simulink model "BMS_V4"  (R2017b)
settings: Solver=FixedStepDiscrete  StartTime=0.0  StopTime=inf  FixedStep=BASETIME  RelTol=1e-3  EnableMultiTasking=on
values from neighbouring files (symbols this model uses):
  AKT_BALANCE = uint16(8)    [BMS_V4_config.m]
  BALANCE = uint16(4)    [BMS_V4_config.m]
  BALANCE_RESISTOR = int32(5)    [BMS_V4_config.m]
  BALANCE_VEC = uint16(8)    [BMS_V4_config.m]
  CELL_SOC = uint16(7)    [BMS_V4_config.m]
  CELL_STATE = uint16(3)    [BMS_V4_config.m]
  CELL_TEMPERATURE = uint16(6)    [BMS_V4_config.m]
  CELL_VOLTAGE = uint16(5)    [BMS_V4_config.m]
  CELLACTBITFIELD = hex2dec('300')    [BMS_V4_config.m]
  CELLDEACTBITFIELD = hex2dec('100')    [BMS_V4_config.m]
  CELLT_BURST = uint16(6)    [BMS_V4_config.m]
  CELLV_BURST = uint16(5)    [BMS_V4_config.m]
  CLK_CYC_timer_1 = 586    [BMS_V4_config.m]
  CLK_CYC_timer_2 = 5860    [BMS_V4_config.m]
  CLK_CYC_timer_3 = 280    [BMS_V4_config.m]
  CLK_CYC_timer_4 = 586*100    (= 58600)    [BMS_V4_config.m]
  CLK_CYC_timer_5 = 5800*2    (= 11600)    [BMS_V4_config.m]
  CLK_CYC_timer_6 = 320    [BMS_V4_config.m]
  CN_CELLS = int32(40*3600)    [BMS_V4_config.m]
  CONTACTOR = uint16(1)    [BMS_V4_config.m]
  CONTACTOR_LOCKED = uint16(0)    [BMS_V4_config.m]
  CONTACTOR_UNLOCKED = uint16(1)    [BMS_V4_config.m]
  DEBUG_SEND_STATES = uint16(hex2dec('01'))    [BMS_V4_config.m]
  DELTA_SOC_BALANCE = int32(5*1e6)    [BMS_V4_config.m]
  DELTA_SOC_BALANCE_OFF = int32(1*1e5)    [BMS_V4_config.m]
  DETERMINE_MODEL_PARAMETER_ACT = uint16(100)    [BMS_V4_config.m]
  DETERMINE_MODEL_PARAMETER_SCC = uint16(101)    [BMS_V4_config.m]
  ERROR = uint16(1)    [BMS_V4_config.m]
  EXTERN_SIGNALS = uint16(1)    [BMS_V4_config.m]
  FREQUENCY_STEPS = uint16([25 50 75 100 150 250 500 750                                      1000 1500 2500 5000 7500                                      10010 10015 10025 10050 10075                                      10100 10150 10250 10500 10750                                      11000 11500])    [BMS_V4_config.m]
  GET_IMAG_PART_MFC = uint16(9)    [BMS_V4_config.m]
  GET_IMAG_PART_MSF = uint16(4)    [BMS_V4_config.m]
  GET_REAL_PART_MFC = uint16(8)    [BMS_V4_config.m]
  GET_REAL_PART_MSF = uint16(3)    [BMS_V4_config.m]
  IMU = uint16(7)    [BMS_V4_config.m]
  IMU_AMP_OFF = uint16(5)    [BMS_V4_config.m]
  IMU_DATA_READ_LOCUS_ACT = uint16(6)    [BMS_V4_config.m]
  IMU_DATA_READ_LOCUS_SCC = uint16(7)    [BMS_V4_config.m]
  IMU_DEBUG = uint16(9)    [BMS_V4_config.m]
  IMU_GET_DATA_MFC = uint16(8)    [BMS_V4_config.m]
  IMU_GET_DATA_MSF = uint16(3)    [BMS_V4_config.m]
  IMU_OFFSET_POLLING = uint16(11)    [BMS_V4_config.m]
  IMU_POLLING = uint16(2)    [BMS_V4_config.m]
  IMU_POWER = uint16(10)    [BMS_V4_config.m]
  IMU_SEND_IMAG = uint16(11)    [BMS_V4_config.m]
  IMU_SEND_REAL = uint16(10)    [BMS_V4_config.m]
  INDEX_IMAGPART = uint16(2)    [BMS_V4_config.m]
  INDEX_REALPART = uint16(1)    [BMS_V4_config.m]
  INFO = uint16(2)    [BMS_V4_config.m]
  INIT_OFFSET_AMPLITUDE = uint16(2)    [BMS_V4_config.m]
  LINE_CURRENT = uint16(3)    [BMS_V4_config.m]
  LINE_CURRENT_CANA = uint16(4)    [BMS_V4_config.m]
  LINE_CURRENT_SWITCH_THRESHOLD = int32(2*1e6)    [BMS_V4_config.m]
  NUM_OF_CELLS = uint16(16)    [BMS_V4_config.m]
  NUM_OF_FREQUENCIES_PSO = uint16(14)    [BMS_V4_config.m]
  NUM_OF_LINES = uint16(1)    [BMS_V4_config.m]
  NUM_OF_PARAMETER = single(5)    [BMS_V4_config.m]
  NUM_OF_SOC_POINTS = uint16(110)    [BMS_V4_config.m]
  P_L_BOUND = single([0.05;0.01;0.1;0.01;0.1])    [BMS_V4_config.m]
  P_U_BOUND = single([0.50;0.20;0.9;0.06;60])    [BMS_V4_config.m]
  PARA_ACT_SEND = uint16(101)    [BMS_V4_config.m]
  PARA_DATA_STORE_ACT = uint16(8)    [BMS_V4_config.m]
  PARA_DATA_STORE_SCC = uint16(9)    [BMS_V4_config.m]
  PARA_SCC_SEND = uint16(102)    [BMS_V4_config.m]
  PARTICLE_INIT = single(create_startparticle(P_L_BOUND,P_U_BOUND,NUM_OF_PARTICLE))    [BMS_V4_config.m]
  POLACT = hex2dec('00000BFF')    [BMS_V4_config.m]
  POLDEACT = hex2dec('000008FF')    [BMS_V4_config.m]
  PSO_PARA_DEBUG = uint16(13)    [BMS_V4_config.m]
  REQUEST_SOC_REF = uint16(1000)    [BMS_V4_config.m]
  SCALE_FACTOR_CH1 = single(0.66666666)    [BMS_V4_config.m]
  SCALE_FACTOR_CH2 = single(0.66666666)    [BMS_V4_config.m]
  SEND_CELL_SOC_ABS = uint16(199)    [BMS_V4_config.m]
  SHUT_DOWN_BALANCE_OFF = uint16(3)    [BMS_V4_config.m]
  SHUT_DOWN_BALANCE_ON = uint16(2)    [BMS_V4_config.m]
  START_IMU_MSL = uint16(3)    [BMS_V4_config.m]
  START_IMU_SCC = uint16(1)    [BMS_V4_config.m]
  SWITCH_IMU_OFF = uint16(2)    [BMS_V4_config.m]
  SWITCH_IMU_ON = uint16(1)    [BMS_V4_config.m]
  SWITCH_IMU_ON_OFF = uint16(4)    [BMS_V4_config.m]
  SYSTEM_DEBUG = uint16(12)    [BMS_V4_config.m]
  TIMEOUT_CANA = uint32(5000)    [BMS_V4_config.m]
  TIMEOUT_GATEWAY = uint32(500)    [BMS_V4_config.m]
  TS_SOC = single(0.010)    [BMS_V4_config.m]
  WARNING = uint16(2)    [BMS_V4_config.m]
libraries: c280xlib x44, c2833xlib x5, simulink x2, c2000lib x1, idelinklib_common x1
(part 3 of 8)

== matlab function BMS_V4/FunctionCall_CANB_RX/handle_cellV_burst/cellV_proceeding ==
  data: msg input; NUM_OF_CELLS parameter; cell_voltages data_store_memory; next_gateway_request data_store_memory; gateway_request data_store_memory; CELLV_BURST parameter
function cellV_proceedng(msg,NUM_OF_CELLS, CELLV_BURST)

global cell_voltages;
global next_gateway_request;
global gateway_request;

x1      = uint16(bitand(uint32(hex2dec('0000FFFF')),msg(1)));
line_nr = uint16(bitand(uint16(hex2dec('00FF')),x1))+uint16(1);
cell_nr = uint16(bitand(uint16(hex2dec('00FF')),bitshift(x1,-8)))+uint16(1);
% cell number and line number starting with zero from Gateway
volt1   = uint16(bitand(uint32(hex2dec('0000FFFF')),bitshift(msg(1),-16)));
volt2   = uint16(bitand(uint32(hex2dec('0000FFFF')),bitshift(msg(2),-0)));
volt3   = uint16(bitand(uint32(hex2dec('0000FFFF')),bitshift(msg(2),-16)));

if (cell_nr + uint16(1)) > NUM_OF_CELLS % last msg with only one voltages
    cell_voltages(cell_nr, line_nr) = uint16(volt1); 
%     gateway_request(CELLV_BURST) = false;
    next_gateway_request=true;
elseif (cell_nr + uint16(2)) > NUM_OF_CELLS % last msg with only two voltages in msg
    cell_voltages(cell_nr, line_nr) = uint16(volt1); 
    cell_voltages(cell_nr+uint16(1),line_nr) = uint16(volt2);
%     gateway_request(CELLV_BURST) = false;
   next_gateway_request=true;
elseif (cell_nr + uint16(3)) > NUM_OF_CELLS % last msg with three voltages
    cell_voltages(cell_nr          , line_nr) = uint16(volt1); 
    cell_voltages(cell_nr+uint16(1), line_nr) = uint16(volt2);
    cell_voltages(cell_nr+uint16(2), line_nr) = uint16(volt3);
%     gateway_request(CELLV_BURST) = false;
    next_gateway_request=true;
else % more msg
    cell_voltages(cell_nr          , line_nr) = uint16(volt1); 
    cell_voltages(cell_nr+uint16(1), line_nr) = uint16(volt2);
    cell_voltages(cell_nr+uint16(2), line_nr) = uint16(volt3);
end

== matlab function BMS_V4/FunctionCalll_CANB_send/Send_gateway_request_control ==
  data: contactor_enable output; CAN_contactor_low output; CAN_contactor_high output; info_enable output; CAN_info_low output; CAN_info_high output; line_current_enable output; CAN_line_current_low output; CAN_line_current_high output; balance_enable output; CAN_balance_low output; CAN_balance_high output; cellV_burst_enable output; CAN_cellV_low output; CAN_cellV_high output; cellT_burst_enable output; CAN_cellT_low output; timer_ms data_store_memory; NUM_OF_CELLS parameter; NUM_OF_LINES parameter; TIMEOUT_GATEWAY parameter; next_gateway_request data_store_memory; gateway_request data_store_memory; CAN_cellT_high output; CONTACTOR parameter; LINE_CURRENT parameter; INFO parameter; CELLV_BURST parameter; CELLT_BURST parameter; BALANCE parameter; contactor_request data_store_memory; SHUT_DOWN_BALANCE_ON parameter; SHUT_DOWN_BALANCE_OFF parameter; EXTERN_SIGNALS parameter; information_mode data_store_memory; imu_CAN_high data_store_memory; imu_CAN_low data_store_memory; control_imu_enable output; CAN_control_imu_low output; CAN_control_imu_high output; IMU parameter; balance_vector data_store_memory; active_balance_enable output; CAN_act_balance_low output; CAN_act_balance_high output; AKT_BALANCE parameter; active_balance_vector data_store_memory; error_state data_store_memory; balance_flag data_store_memory; POLDEACT parameter; CELLACTBITFIELD parameter; CELLDEACTBITFIELD parameter; POLACT parameter
function [contactor_enable, CAN_contactor_low, CAN_contactor_high,...
  info_enable, CAN_info_low, CAN_info_high,...
  line_current_enable,CAN_line_current_low, CAN_line_current_high,...
  balance_enable, CAN_balance_low, CAN_balance_high,...
  cellV_burst_enable, CAN_cellV_low, CAN_cellV_high,...
  cellT_burst_enable,CAN_cellT_low, CAN_cellT_high,...
  control_imu_enable,CAN_control_imu_low, CAN_control_imu_high,...
  active_balance_enable, CAN_act_balance_low, CAN_act_balance_high]...
 = Send_gateway_request_control...
    (NUM_OF_CELLS, NUM_OF_LINES , TIMEOUT_GATEWAY, CONTACTOR,...
    LINE_CURRENT, INFO,CELLV_BURST, CELLT_BURST, BALANCE,...
    SHUT_DOWN_BALANCE_ON, SHUT_DOWN_BALANCE_OFF, EXTERN_SIGNALS,IMU, AKT_BALANCE, POLDEACT, CELLACTBITFIELD, CELLDEACTBITFIELD, POLACT)

global next_gateway_request;
global gateway_request;
global timer_ms;
%global contactor_unlocked;
global contactor_request;
global information_mode;
global imu_CAN_high;
global imu_CAN_low;
global balance_vector;
global balance_flag;
global active_balance_vector;
global error_state;

persistent timer_old;
if isempty(timer_old)
    timer_old = uint32(0);
end


CAN_cellV_high = uint32(0);
CAN_cellV_low = uint32(0);
CAN_cellT_high = uint32(0);
CAN_cellT_low = uint32(0);
CAN_line_current_high = uint32(0);
CAN_line_current_low = uint32(0);

CAN_info_high = uint32(0);
CAN_info_low = uint32(0);
CAN_contactor_high = uint32(0);
CAN_contactor_low = uint32(0);
CAN_balance_high = uint32(0);
CAN_balance_low = uint32(0);
CAN_control_imu_low = uint32(0);
CAN_control_imu_high = uint32(0);
CAN_act_balance_low= uint32(0);
CAN_act_balance_high= uint32(0);

control_imu_enable =false;
cellV_burst_enable = false;
cellT_burst_enable = false;
line_current_enable = false;
contactor_enable = false;
info_enable = false;
balance_enable = false;
active_balance_enable= false;


if(next_gateway_request == true)                                                   
    timer_old = timer_ms;
    if (gateway_request(CONTACTOR) == true)
        % contactor
        next_gateway_request = false;
        if contactor_request == true
            CAN_contactor_low = uint32(1);      % contactor on
        else
            CAN_contactor_low = uint32(0);      % contactor off
        end
        CAN_contactor_high = uint32(0); 
        contactor_enable = true;
       gateway_request(CONTACTOR) = false;
        
        
    elseif (gateway_request(INFO) == true)                                
        % information
        next_gateway_request = false;
        if (information_mode == SHUT_DOWN_BALANCE_OFF)
            %Shut down with balance off
            CAN_info_low = uint32(3);
            CAN_info_high = uint32(0);
        elseif(information_mode == SHUT_DOWN_BALANCE_ON)
            %Shut down with balance on
            CAN_info_low = uint32(4);
            CAN_info_high = uint32(0);
        elseif(information_mode == EXTERN_SIGNALS)
            % request extern signals                         
            CAN_info_low = uint32(1);
            CAN_info_high = uint32(0);
        end
        info_enable = true;   
       gateway_request(INFO) = false;
    
    elseif (gateway_request(LINE_CURRENT) == true)
       % line current
       next_gateway_request = false;
       line_nr = uint32(0);
       CAN_line_current_low = uint32(line_nr);
       CAN_line_current_high = uint32(0);
       line_current_enable = true;
      gateway_request(LINE_CURRENT) = false;   
      
    elseif (gateway_request(BALANCE) == true)
       % balance   
       line_nr = uint32(0);
       CAN_balance_low = uint32(line_nr);
       for i = 1:1:NUM_OF_CELLS
           CAN_balance_low = uint32(bitor(CAN_balance_low,uint32...
           (bitshift(uint32(balance_vector(i)),15+i))));
       end
       CAN_balance_high_ = uint32(0);
       balance_enable = true;       
      gateway_request(BALANCE) = false;        

     elseif (gateway_request(CELLV_BURST) == true)
         % voltage burst
          next_gateway_request = false;
          line_nr=uint32(0);          
          CAN_cellV_low = uint32(line_nr);
          CAN_cellV_high  = uint32(0);
          cellV_burst_enable = true;
         gateway_request(CELLV_BURST) = false;
        
    elseif (gateway_request(CELLT_BURST) == true)
        % temperatur burst
         next_gateway_request = false;
         line_nr=uint32(0);
         CAN_cellT_low = uint32(line_nr);
         CAN_cellT_high  = uint32(0);
         cellT_burst_enable = true;
        gateway_request(CELLT_BURST) = false;
         
    elseif (gateway_request(IMU) == true)
        % control IMU
         next_gateway_request = false;
         line_nr=uint32(0);
         CAN_control_imu_low = imu_CAN_low;
         CAN_control_imu_high  = imu_CAN_high;
         control_imu_enable = true;
        gateway_request(IMU) = false;
        
    elseif (gateway_request(AKT_BALANCE)== true) %CAN-Messages for the Active-AuxSup-Balancing-Charger
        
        next_gateway_request = false;
        gateway_request(AKT_BALANCE)= false;
     
       % balance_need =   max(active_balance_vector(:,1)); %Balance need
        balance_on =    max(active_balance_vector(:,3)); %Balance is on
        changes = active_balance_vector(:,1) ~= active_balance_vector(:,3);
        changes_need = max(changes);
       
        %Deaktivation of all the Balancing if an error occours or the the
        %Master leaves the states where balancing is allowed
        if   ((error_state(2)> 0 )||((balance_flag == 0)&&( balance_on>0)));
            %Polling with deactivation
            CAN_act_balance_low= uint32(POLDEACT);
            CAN_act_balance_high= uint32(0);
            active_balance_enable = true;
           
        %Change the status of a single cell if the need and the
        %activated states differs
        elseif (balance_flag == 1)&&(changes_need > 0)
            %Change Cell states
            
           
           for k=1:1:NUM_OF_CELLS
            if active_balance_vector(k,1) ~= active_balance_vector(k,3)
                cellnumb = uint32(k);
                break;
            else
                cellnumb = uint32(0);
            end
           end
           
           
           cellnumbshift = uint32(bitshift(cellnumb,0));
           % cell need activation
           if active_balance_vector(cellnumb,1) > active_balance_vector(cellnumb,3)
               chargeneed = uint32(active_balance_vector(cellnumb,2));
               bitfield = uint32(CELLACTBITFIELD);
               active_balance_vector(cellnumb,3)=uint32(1); 
           else
              chargeneed = uint32(0);
              bitfield = uint32(CELLDEACTBITFIELD);
              active_balance_vector(cellnumb,3)=uint32(0);
             
           end  
                CAN_act_balance_low= uint32(bitor(cellnumbshift,bitfield));
                CAN_act_balance_high= uint32(chargeneed);
                active_balance_enable = true;
        %Standard polling msg while balancing is allowed to get the 
        %actual cell statuses (activation and progress)
        elseif (balance_flag == 1)&&(changes_need <= 0)
            %Polling No Cell Changes
            
            CAN_act_balance_low= uint32(POLACT);
            CAN_act_balance_high= uint32(0);
            active_balance_enable = true;
           
            
        %Standard polling msg while balancing is prohibitet as a heart-
        %beat and to confirm the deactivation
        else
         %Polling with deactivation
            CAN_act_balance_low= uint32(POLDEACT);
            CAN_act_balance_high= uint32(0);
            active_balance_enable = true;
         
        end
    
    end
        
    
else
    
    if((timer_ms-timer_old) > TIMEOUT_GATEWAY)
       next_gateway_request = true; 
        timer_old = timer_ms-uint32(1);
    end
end

== stateflow chart BMS_V4/FunctionCall_timer_1/Timing_control ==
  state Timing_control_CANB_gateway_request [parallel]
    settings: executionOrder=3
    state Voltage_timing [parallel]
      settings: executionOrder=1
      state cell_voltage_request
      state cell_voltage_request_set
        entry:
        gateway_request[CELLV_BURST-uint16(1)]=true;
      (default) -> cell_voltage_request
      cell_voltage_request -> cell_voltage_request_set : after(TIMER_VOLTAGE_REQUEST,sec)
      cell_voltage_request_set -> cell_voltage_request
    state Info_timing [parallel]
      settings: executionOrder=2
      state info_request
      state info_request_set
        entry:
        gateway_request[INFO-uint16(1)]=true;
      (default) -> info_request
      info_request -> info_request_set : after(TIMER_INFO_REQUEST,sec)
      info_request_set -> info_request
    state Temperature_timing [parallel]
      settings: executionOrder=3
      state cell_temperature_request
      state cell_temperature_request_set
        entry:
        gateway_request[CELLT_BURST-uint16(1)]=true;
      (default) -> cell_temperature_request
      cell_temperature_request -> cell_temperature_request_set : after(TIMER_TEMPERATURE_REQUEST,sec)
      cell_temperature_request_set -> cell_temperature_request
    state Line_current_timing [parallel] [commented out]
      state line_current_request [commented out]
      state line_current_request_set [commented out]
        entry:
        gateway_request[LINE_CURRENT-uint16(1)]=true;
      (default) -> line_current_request [commented out]
      line_current_request -> line_current_request_set [commented out] : after(TIMER_LINE_CURRENT_REQUEST,sec)
      line_current_request_set -> line_current_request [commented out]
    state Balancing_timing1 [parallel]
      settings: executionOrder=4
      state activ_balancing_request
      state activ_balancing_request_set1
        entry:
        gateway_request[AKT_BALANCE-uint16(1)]=true;
      (default) -> activ_balancing_request
      activ_balancing_request -> activ_balancing_request_set1 : after(TIMER_ACTIVE_BALANCE_REQUEST,sec)
      activ_balancing_request_set1 -> activ_balancing_request
  state Timing_control_CANA_send_data [parallel]
    settings: executionOrder=1
    state Voltage_timing [parallel]
      settings: executionOrder=1
      state Send_cell_voltage
      state Send_cell_voltage_set
        entry:
        CANA_send_data[CELL_VOLTAGE-uint16(1)]=true;
      (default) -> Send_cell_voltage
      Send_cell_voltage -> Send_cell_voltage_set : after(TIMER_CELL_VOLTAGE,sec)
          | [ imu_send_meas_data == false ]
      Send_cell_voltage_set -> Send_cell_voltage
    state SOC_timing [parallel]
      settings: executionOrder=2
      state Send_soc
      state Send_soc_set
        entry:
        CANA_send_data[CELL_SOC-uint16(1)]=true;
      (default) -> Send_soc
      Send_soc -> Send_soc_set : after(TIMER_CELL_SOC,sec)
          | [ imu_send_meas_data == false ]
      Send_soc_set -> Send_soc
    state Temperature_timing [parallel]
      settings: executionOrder=3
      state Send_cell_temperature
      state Send_cell_temperature_set
        entry:
        CANA_send_data[CELL_TEMPERATURE-uint16(1)]=true;
      (default) -> Send_cell_temperature
      Send_cell_temperature -> Send_cell_temperature_set : after(TIMER_CELL_TEMPERATURE,sec)
          | [ imu_send_meas_data == false ]
      Send_cell_temperature_set -> Send_cell_temperature
    state Line_current_timing [parallel]
      settings: executionOrder=4
      state Send_line_current
      state Send_line_current_set
        entry:
        CANA_send_data[LINE_CURRENT_CANA-uint16(1)]=true;
      (default) -> Send_line_current
      Send_line_current -> Send_line_current_set : after(TIMER_LINE_CURRENT,sec)
          | [ imu_send_meas_data == false ]
      Send_line_current_set -> Send_line_current
    state Cell_states_timing [parallel]
      settings: executionOrder=6
      state Send_cell_states
      state Send_cell_states_set
        entry:
        CANA_send_data[CELL_STATE-uint16(1)]=true;
      (default) -> Send_cell_states
      Send_cell_states -> Send_cell_states_set : after(TIMER_CELL_STATES,sec)
          | [ imu_send_meas_data == false ]
      Send_cell_states_set -> Send_cell_states
    state IMU_debug_timing [parallel]
      settings: executionOrder=5
      state Send_imu_debug
      state Send_imu_set
        entry:
        CANA_send_data[IMU_DEBUG-uint16(1)]=true;
      (default) -> Send_imu_debug
      Send_imu_debug -> Send_imu_set : after(TIMER_IMU_DEBUG,sec)
          | [ imu_send_meas_data == false ]
      Send_imu_set -> Send_imu_debug
    state Balance_vector_timing [parallel]
      settings: executionOrder=7
      state Send_balance_vector
      state Send_balance_vector_set
        entry:
        CANA_send_data[BALANCE_VEC-uint16(1)]=true;
      (default) -> Send_balance_vector
      Send_balance_vector -> Send_balance_vector_set : after(TIMER_BALANCE_VECTOR,sec)
          | [ imu_send_meas_data == false ]
      Send_balance_vector_set -> Send_balance_vector
    state system_debug_timing [parallel]
      settings: executionOrder=8
      state Send_system_debug
      state Send_system_debug_set
        entry:
        system_debug_request = SEND_CELL_SOC_ABS;
        CANA_send_data[SYSTEM_DEBUG-uint16(1)]=true;
      (default) -> Send_system_debug
      Send_system_debug -> Send_system_debug_set : after(TIMER_CELL_SOC_ABS,sec)
          | [ imu_send_meas_data == false ]
      Send_system_debug_set -> Send_system_debug
  state Timing_control_system [parallel]
    settings: executionOrder=2
    state safe_soc_mram [parallel]
      settings: executionOrder=1
      state safe_mram_soc_request
      state safe_mram_soc_set
        entry:
        mram_command[SOC_CC_STORE-uint16(1)] = true;
        mram_command[SOC_ABS_STORE-uint16(1)] = true
      (default) -> safe_mram_soc_request
      safe_mram_soc_request -> safe_mram_soc_set : after(TIMER_SAFE_SOC_MRAM_REQUEST,sec)
      safe_mram_soc_set -> safe_mram_soc_request : [(mram_command[SOC_CC_STORE-uint16(1)] == true) &&...
          |  (mram_command[SOC_ABS_STORE-uint16(1)] == true)]
  data: TIMER_VOLTAGE_REQUEST parameter; TIMER_TEMPERATURE_REQUEST parameter; TIMER_INFO_REQUEST parameter; TIMER_LINE_CURRENT_REQUEST parameter; gateway_request data_store_memory; CELLV_BURST parameter; INFO parameter; LINE_CURRENT parameter; CELLT_BURST parameter; CANA_send_data data_store_memory; TIMER_CELL_VOLTAGE parameter; TIMER_CELL_TEMPERATURE parameter; TIMER_CELL_SOC parameter; TIMER_LINE_CURRENT parameter; LINE_CURRENT_CANA parameter; CELL_VOLTAGE parameter; CELL_TEMPERATURE parameter; CELL_SOC parameter; imu_send_meas_data data_store_memory; TIMER_IMU_DEBUG parameter; IMU_DEBUG parameter; TIMER_CELL_STATES parameter; CELL_STATE parameter; TIMER_SAFE_SOC_MRAM_REQUEST parameter; SOC_CC_STORE parameter; mram_command data_store_memory; TIMER_BALANCE_VECTOR parameter; BALANCE_VEC parameter; SOC_ABS_STORE parameter; TIMER_CELL_SOC_ABS parameter; system_debug_request data_store_memory; SEND_CELL_SOC_ABS parameter; SYSTEM_DEBUG parameter; AKT_BALANCE parameter; TIMER_ACTIVE_BALANCE_REQUEST parameter

== matlab function BMS_V4/FunctionCall_CANB_RX/handle_cellT_burst/cellT_proceeding ==
  data: msg input; NUM_OF_CELLS parameter; next_gateway_request data_store_memory; cell_temperatures data_store_memory; gateway_request data_store_memory; CELLT_BURST parameter
function cellT_proceedng(msg,NUM_OF_CELLS, CELLT_BURST)

global cell_temperatures;
global next_gateway_request;
global gateway_request;

x1      = uint16(bitand(uint32(hex2dec('0000FFFF')),msg(1)));
line_nr = uint16(bitand(uint16(hex2dec('00FF')),x1))+uint16(1);
cell_nr = uint16(bitand(uint16(hex2dec('00FF')),bitshift(x1,-8)))+uint16(1);
% cell number and line number starting with zero from Gateway
temp1   = uint16(bitand(uint32(hex2dec('0000FFFF')),bitshift(msg(1),-16)));
temp2   = uint16(bitand(uint32(hex2dec('0000FFFF')),bitshift(msg(2),-0)));
temp3   = uint16(bitand(uint32(hex2dec('0000FFFF')),bitshift(msg(2),-16)));

temp1_v = single(temp1)/single(1e4);
temp2_v = single(temp2)/single(1e4);
temp3_v = single(temp3)/single(1e4);

temp1 = (((single(5)/temp1_v)-single(1))*single(259.7))-single(259.7);
temp2 = (((single(5)/temp2_v)-single(1))*single(259.7))-single(259.7);
temp3 = (((single(5)/temp3_v)-single(1))*single(259.7))-single(259.7);

if (cell_nr + uint16(1)) > NUM_OF_CELLS % last msg with only one temp
    cell_temperatures(cell_nr ,line_nr) = int16(temp1*single(100));
%     gateway_request(CELLT_BURST) = false;
    next_gateway_request=true;
elseif (cell_nr + uint16(2)) > NUM_OF_CELLS % last msg with only two temp
    cell_temperatures(cell_nr,line_nr) = int16(temp1*single(100)); 
    cell_temperatures(cell_nr+uint16(1),line_nr) = int16(temp2*single(100));
%     gateway_request(CELLT_BURST) = false;
    next_gateway_request=true;
elseif (cell_nr + uint16(3)) > NUM_OF_CELLS % last msg with three temp
    cell_temperatures(cell_nr,line_nr) = int16(temp1*single(100)); 
    cell_temperatures(cell_nr+uint16(1),line_nr) = int16(temp2*single(100));
    cell_temperatures(cell_nr+uint16(2),line_nr) = int16(temp3*single(100));
%     gateway_request(CELLT_BURST) = false;
    next_gateway_request=true;
else % more msg
    cell_temperatures(cell_nr,line_nr) = int16(temp1*single(100)); 
    cell_temperatures(cell_nr+uint16(1),line_nr) = int16(temp2*single(100));
    cell_temperatures(cell_nr+uint16(2),line_nr) = int16(temp3*single(100));
end

== matlab function BMS_V4/FunctionCall_CANB_RX/handle_line_current/line_current_proceeding ==
  data: msg input; next_gateway_request data_store_memory; current_CH1 output; current_CH2 output; line_no output; activate_current_correction data_store_memory; correction_current_CH1 data_store_memory; correction_current_CH2 data_store_memory
function [current_CH1, current_CH2,line_no]=line_current_proceedng(msg)

global activate_current_correction;
global correction_current_CH1;
global correction_current_CH2;


line_no = uint16(bitand(uint32(hex2dec('000000FF')),msg(1)))+uint16(1);

current_V_CH1 = uint16(bitand(uint32(hex2dec('0000FFFF')),...
    bitshift(msg(1),-8)));

current_V_CH2 = uint16(bitor(bitand(uint32(hex2dec('000000FF')),...
    bitshift(msg(1),-24)),bitand(uint32(hex2dec('0000FF00')),...
    bitshift(msg(2),8))));

if(activate_current_correction == true)
    
    correction_current_CH1 = single(current_V_CH1)/single(1e4);
    correction_current_CH2 = single(current_V_CH2)/single(1e4);
    activate_current_correction = false;
    
end

current_CH1 = current_V_CH1;
current_CH2 = current_V_CH2;

== matlab function BMS_V4/FunctionCall_CANB_RX/handle_line_current/save_current ==
  data: current input; line_no input; next_gateway_request data_store_memory; line_currents data_store_memory; LINE_CURRENT parameter; gateway_request data_store_memory
function save_current(current,line_no, LINE_CURRENT)
% Datenempfang über CAN

global line_currents;
global next_gateway_request;
global gateway_request;

line_currents(line_no)=current;
%line_currents(line_no)=int32(0);

gateway_request(LINE_CURRENT) = false;
next_gateway_request = true;

== matlab function BMS_V4/FunctionCall_CANB_RX/handle_info/info_proceeding ==
  data: msg input; next_gateway_request data_store_memory; information_code data_store_memory; EXTERN_SIGNALS parameter; gateway_request data_store_memory; INFO parameter
function info_proceedng(msg, EXTERN_SIGNALS, INFO)

global information_code;
global next_gateway_request;
global gateway_request;

code = uint16(bitand(uint32(hex2dec('000000FF')),msg(1)));
msg  = uint16(bitand(uint32(hex2dec('000000FF')),bitshift(msg(1),-8)));

if(code == EXTERN_SIGNALS)
    information_code=uint16(msg);
end

% gateway_request(INFO) = false;
next_gateway_request=true;

== matlab function BMS_V4/FunctionCall_CANB_RX/handle_contactor/contactor_proceeding ==
  data: msg input; next_gateway_request data_store_memory; contactor_unlocked data_store_memory; CONTACTOR_UNLOCKED parameter; CONTACTOR_LOCKED parameter; gateway_request data_store_memory; CONTACTOR parameter
function contactor_proceedng(msg,CONTACTOR_UNLOCKED,CONTACTOR_LOCKED, CONTACTOR)

global contactor_unlocked;
global next_gateway_request;
global gateway_request;

code = uint16(bitand(uint32(hex2dec('000000FF')),msg(1)));
if code == CONTACTOR_UNLOCKED
    contactor_unlocked=true;
elseif code == CONTACTOR_LOCKED
    contactor_unlocked=false;
end

% gateway_request(CONTACTOR) = false;
next_gateway_request=true;

== matlab function BMS_V4/FunctionCall_CANB_RX/handle_balance/balance_proceeding ==
  data: msg input; next_gateway_request data_store_memory; gateway_request data_store_memory; BALANCE parameter
function balance_proceedng(msg, BALANCE)

global next_gateway_request;
global gateway_request;
%t.b.d
%code = uint16(bitand(uint32(hex2dec('000000FF')),msg(1)));

% gateway_request(BALANCE) = false;  
next_gateway_request=true;
